simulink model "scara_2015a_dSpace"  (R2018b)
settings: Solver=ode1  StartTime=0.0  StopTime=inf  FixedStep=0.001  RelTol=1e-3
PostLoadFcn:
  | , if any(exist('dsrtsu_mdlpostloadfcn', 'file') == [2, 3, 6]), try dsrtsu_mdlpostloadfcn('Execute', bdroot); catch fprintf('Error in PostLoadFcn (dsrtsu_mdlpostloadfcn) for model "%s":\n %s\n', bdroot, lasterr); end, end,
libraries: rtilib1104 x9, simulink x5, simulink_extras x4
settings Model: DSRTSU_INTERNAL_RTI_VER=460  DSRTSU_INTERNAL_RTI_TYPE=rti1104  DSRTSU_INTERNAL_RTIFPGA=50  Creator=Bartlomiej Mroz  LastModifiedBy=Bartlomiej Mroz
settings OptimizationCC: BlockReduction=off  BooleanDataType=off  LifeSpan=inf
settings DebuggingCC: SFExecutionAtInitializationDiag=none
settings HardwareCC: ProdBitPerSizeT=32  ProdBitPerPtrDiffT=32  ProdEndianess=BigEndian  ProdWordSize=32  ProdHWDeviceType=Generic->Custom  TargetIntDivRoundTo=Zero  TargetEndianess=BigEndian  TargetHWDeviceType=Generic->Custom
settings RTWCC: SystemTargetFile=rti1104.tlc  MakeCommand=make_rti  TemplateMakefile=rti1104.tmf  Description=dSPACE DS1104 Hardware Platform
settings CodeAppCC: StateflowObjectComments=on
settings STFCustomTargetCC: ParMdlRefBuildCompliant=on  GeneratePreprocessorConditionals=Disable all  GRTInterface=on  SystemTargetFile=rti1104.tlc
settings GRTTargetCC: TargetLangStandard=C89/C90 (ANSI)  CompOptLevelCompliant=off  ConcurrentExecutionCompliant=off  GeneratePreprocessorConditionals=Disable all  CombineOutputUpdateFcns=off  MatFileLogging=off  CPPClassGenCompliant=off  GRTInterface=on  UseToolchainInfoCompliant=off  ExtModeMexFile=noextcomm

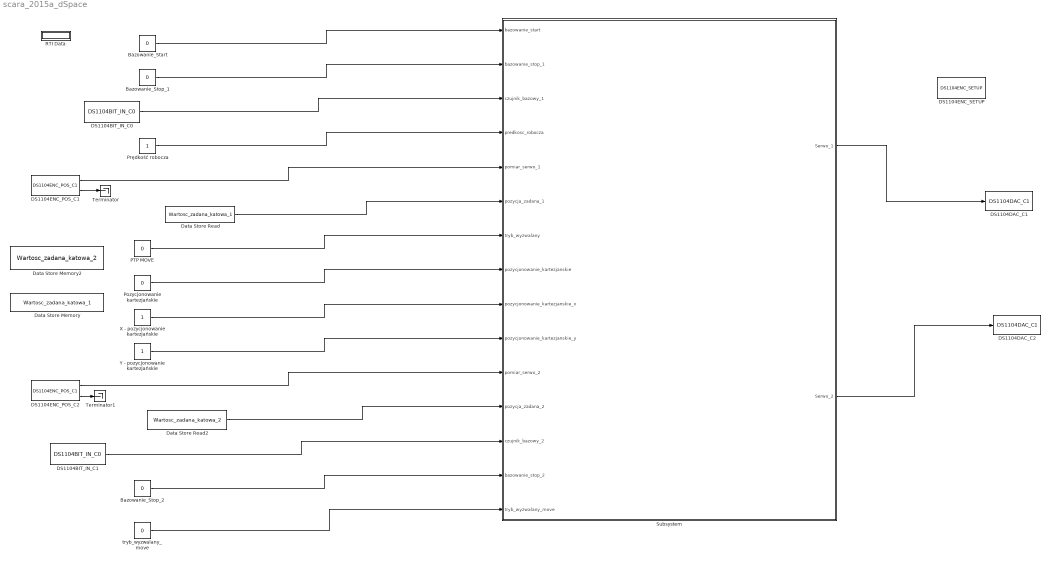
== system scara_2015a_dSpace ==
  " Bazowanie_Stop_1" : Constant  Value=0
  " Bazowanie_Stop_2" : Constant  Value=0
  " tryb_wyzwalany_move" : Constant  Value=0
  Bazowanie_Start : Constant  Value=0
  DS1104BIT_IN_C0 : rtilib1104/DS1104 MASTER PPC/DS1104BIT_IN_C0  ChannelNo=0  Reserved1=[]  Reserved2=[]  Reserved3=[]  Reserved4=[]  DialogFcn=gui1104bit_in  UnitName={'DS1104BIT_IN_C'}  UnitValues={ 0 }  DSProperties=struct('RTI',struct('Version',uint32(1),'BlockType',struct('isSLSource',uint8(1),'isSLSink',uint8(0),'isHWSource',uint8(1),'isHWSink',uint8(0),'isSetup',uint8(0),'isInline',uint8(1),'isNonInline',uint8(0),'isInterrupt',uint8(0),'isChannelwise',uint8(1)),'IOBoardType','DS1104MASTER','UnitType','BIT','Identifier','BITINCH','DialogType','ML','BlockSet','NONE','SlaveProcessor','NONE'))
  DS1104BIT_IN_C1 : rtilib1104/DS1104 MASTER PPC/DS1104BIT_IN_C0  ChannelNo=1  Reserved1=[]  Reserved2=[]  Reserved3=[]  Reserved4=[]  DialogFcn=gui1104bit_in  UnitName={'DS1104BIT_IN_C'}  UnitValues={1}  DSProperties=struct('RTI',struct('Version',uint32(1),'BlockType',struct('isSLSource',uint8(1),'isSLSink',uint8(0),'isHWSource',uint8(1),'isHWSink',uint8(0),'isSetup',uint8(0),'isInline',uint8(1),'isNonInline',uint8(0),'isInterrupt',uint8(0),'isChannelwise',uint8(1)),'IOBoardType','DS1104MASTER','UnitType','BIT','Identifier','BITINCH','DialogType','ML','BlockSet','NONE','SlaveProcessor','NONE'))
  DS1104DAC_C1 : rtilib1104/DS1104 MASTER PPC/DS1104DAC_C1  ChannelNo=1  InitValue=0  TermMode=1  TermValue=0  Reserved1=[]  Reserved2=[]  Reserved3=[]  Reserved4=[]  DialogFcn=gui1104dac  UnitName={ 'DS1104DAC_C'}  UnitValues={ 1 }  DSProperties=struct('RTI',struct('Version',uint32(1),'BlockType',struct('isSLSource',uint8(0),'isSLSink',uint8(1),'isHWSource',uint8(0),'isHWSink',uint8(1),'isSetup',uint8(0),'isInline',uint8(1),'isNonInline',uint8(0),'isInterrupt',uint8(0),'isChannelwise',uint8(1)),'IOBoardType','DS1104MASTER','UnitType','DAC','Identifier','DAC','DialogType','ML','BlockSet','NONE','SlaveProcessor','NONE'))
  DS1104DAC_C2 : rtilib1104/DS1104 MASTER PPC/DS1104DAC_C1  ChannelNo=2  InitValue=0  TermMode=1  TermValue=0  Reserved1=[]  Reserved2=[]  Reserved3=[]  Reserved4=[]  DialogFcn=gui1104dac  UnitName={ 'DS1104DAC_C'}  UnitValues={2}  DSProperties=struct('RTI',struct('Version',uint32(1),'BlockType',struct('isSLSource',uint8(0),'isSLSink',uint8(1),'isHWSource',uint8(0),'isHWSink',uint8(1),'isSetup',uint8(0),'isInline',uint8(1),'isNonInline',uint8(0),'isInterrupt',uint8(0),'isChannelwise',uint8(1)),'IOBoardType','DS1104MASTER','UnitType','DAC','Identifier','DAC','DialogType','ML','BlockSet','NONE','SlaveProcessor','NONE'))
  DS1104ENC_POS_C1 : rtilib1104/DS1104 MASTER PPC/DS1104ENC_POS_C1  ChannelNo=1  PosValue=0  Reserved1=[]  Reserved2=[]  Reserved3=[]  Reserved4=[]  DialogFcn=gui1104enc_pos  UnitName={'DS1104ENC_POS_C'}  UnitValues={ 1 }  DSProperties=struct('RTI',struct('Version',uint32(1),'BlockType',struct('isSLSource',uint8(1),'isSLSink',uint8(0),'isHWSource',uint8(1),'isHWSink',uint8(0),'isSetup',uint8(0),'isInline',uint8(1),'isNonInline',uint8(0),'isInterrupt',uint8(0),'isChannelwise',uint8(1)),'IOBoardType','DS1104MASTER','UnitType','ENC','Identifier','ENCPOSCH','DialogType','ML','BlockSet','NONE','SlaveProcessor','NONE'))
  DS1104ENC_POS_C2 : rtilib1104/DS1104 MASTER PPC/DS1104ENC_POS_C1  ChannelNo=2  PosValue=0  Reserved1=[]  Reserved2=[]  Reserved3=[]  Reserved4=[]  DialogFcn=gui1104enc_pos  UnitName={'DS1104ENC_POS_C'}  UnitValues={2}  DSProperties=struct('RTI',struct('Version',uint32(1),'BlockType',struct('isSLSource',uint8(1),'isSLSink',uint8(0),'isHWSource',uint8(1),'isHWSink',uint8(0),'isSetup',uint8(0),'isInline',uint8(1),'isNonInline',uint8(0),'isInterrupt',uint8(0),'isChannelwise',uint8(1)),'IOBoardType','DS1104MASTER','UnitType','ENC','Identifier','ENCPOSCH','DialogType','ML','BlockSet','NONE','SlaveProcessor','NONE'))
  DS1104ENC_SETUP : rtilib1104/DS1104 MASTER PPC/DS1104ENC_SETUP  Reserved1=[]  Reserved2=[]  Reserved3=[]  Reserved4=[]  DialogFcn=gui1104enc_setup  UnitName={'DS1104ENC_SETUP'}  UnitValues={ [] }  DSProperties=struct('RTI',struct('Version',uint32(1),'BlockType',struct('isSLSource',uint8(0),'isSLSink',uint8(0),'isHWSource',uint8(0),'isHWSink',uint8(0),'isSetup',uint8(0),'isInline',uint8(1),'isNonInline',uint8(0),'isInterrupt',uint8(0),'isChannelwise',uint8(0)),'IOBoardType','DS1104MASTER','UnitType','ENC','Identifier','ENCSETUP','DialogType','ML','BlockSet','NONE','SlaveProcessor','NONE'))
      settings: SignalType=[0 0]
  Data Store Memory : DataStoreMemory  DataStoreName=Wartosc_zadana_katowa_1  ReadBeforeWriteMsg=warning  WriteAfterWriteMsg=warning  WriteAfterReadMsg=warning  ShowAdditionalParam=off
  Data Store Memory2 : DataStoreMemory  DataStoreName=Wartosc_zadana_katowa_2  ReadBeforeWriteMsg=warning  WriteAfterWriteMsg=warning  WriteAfterReadMsg=warning  ShowAdditionalParam=off
  Data Store Read : DataStoreRead  DataStoreName=Wartosc_zadana_katowa_1
  Data Store Read2 : DataStoreRead  DataStoreName=Wartosc_zadana_katowa_2
  PTP MOVE : Constant  Value=0
  "Pozycjonowanie kartezjańskie " : Constant  Value=0
  Prędkość robocza : Constant
  RTI Data : Subsystem  Tag=struct('RTIDataServer',struct('RTIDataServerVs','2','RTIModelDescription','struct(''main'',''scara_2015a'',''sub'','''',''isMp'',0)'))  LoadFcn="if exist('rtidc'), try,  rtidc('DataHostBlockClbLoad', gcbh); catch, disp(['Warning: ''LoadFcn'' for RTI Data block failed: ' lasterr]); end, end,"  mask(RTI_DATA_HOST){}
      mask help:
      | RTI Data Block.
      | This block is used by RTI to store internal model-dependent data.
      | Please keep this block on the root level of the model. Deleting this block will result in data loss.
      |
      | NEVER DELETE OR COPY THIS BLOCK!
      settings: CopyFcn="if exist('rtidc'), try,  rtidc('DataHostBlockClbCopy', gcbh); catch, disp(['Warning: ''CopyFcn'' for RTI Data block failed: ' lasterr]); end, end,"  DeleteFcn="if exist('rtidc'), try,  rtidc('DataHostBlockClbDelete', gcbh); catch, disp(['Warning: ''DeleteFcn'' for RTI Data block failed: ' lasterr]); end, end,"  ModelCloseFcn="if exist('rtidc'), try,  rtidc('DataHostBlockClbModelClose', gcbh); catch, disp(['Warning: ''ModelCloseFcn'' for RTI Data block failed: ' lasterr]); end, end,"  PreSaveFcn="if exist('rtidc'), try,  rtidc('DataHostBlockClbPreSave', gcbh); catch, disp(['Warning: ''PreSaveFcn'' for RTI Data block failed: ' lasterr]); end, end,"  PostSaveFcn="if exist('rtidc'), try,  rtidc('DataHostBlockClbPostSave', gcbh); catch, disp(['Warning: ''PostSaveFcn'' for RTI Data block failed: ' lasterr]); end, end,"  NameChangeFcn="if exist('rtidc'), try,  rtidc('DataHostBlockClbNameChange', gcbh); catch, disp(['Warning: ''NameChangeFcn'' for RTI Data block failed: ' lasterr]); end, end,"
      mask Help:
      | RTI Data Block.
      | This block is used by RTI to store internal model-dependent data.
      | Please keep this block on the root level of the model. Deleting this block will result in data loss.
      | 
      | NEVER DELETE OR COPY THIS BLOCK!
      mask Display:
      | text(0.5, 0.5, 'RTI Data', 'HorizontalAlignment', 'center');
      | plot([1 0]);
  Subsystem : Subsystem
  Terminator : Terminator
  Terminator1 : Terminator
  X - pozycjonowanie kartezjańskie : Constant
  Y - pozycjonowanie kartezjańskie : Constant
  wires:
  Bazowanie_Start/1 -> Subsystem/1(bazowanie_start)
  " Bazowanie_Stop_1"/1 -> Subsystem/2(bazowanie_stop_1)
  DS1104BIT_IN_C0/1 -> Subsystem/3(czujnik_bazowy_1)
  Prędkość robocza/1 -> Subsystem/4(predkosc_robocza)
  DS1104ENC_POS_C1/1 -> Subsystem/5(pomiar_serwo_1)
  Data Store Read/1 -> Subsystem/6(pozycja_zadana_1)
  PTP MOVE/1 -> Subsystem/7(tryb_wyzwalany)
  "Pozycjonowanie kartezjańskie "/1 -> Subsystem/8(pozycjonowanie_kartezjanskie)
  X - pozycjonowanie kartezjańskie/1 -> Subsystem/9(pozycjonowanie_kartezjanskie_x)
  Y - pozycjonowanie kartezjańskie/1 -> Subsystem/10(pozycjonowanie_kartezjanskie_y)
  DS1104ENC_POS_C2/1 -> Subsystem/11(pomiar_serwo_2)
  Data Store Read2/1 -> Subsystem/12(pozycja_zadana_2)
  DS1104BIT_IN_C1/1 -> Subsystem/13(czujnik_bazowy_2)
  Subsystem/1(Serwo_1) -> DS1104DAC_C1/1
  Subsystem/2(Serwo_2) -> DS1104DAC_C2/1
  DS1104ENC_POS_C1/2 -> Terminator/1
  DS1104ENC_POS_C2/2 -> Terminator1/1
  " Bazowanie_Stop_2"/1 -> Subsystem/14(bazowanie_stop_2)
  " tryb_wyzwalany_move"/1 -> Subsystem/15(tryb_wyzwalany_move)

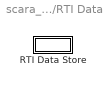
== system scara_2015a_dSpace/RTI Data ==
  RTI Data Store : Subsystem  Tag="struct('private',struct('version',struct('dsVer',uint32(2),'dsVerCreation',uint32(2),'RTI',struct('ver','7.4','type','RTI1104')),'access',struct('type','Model','isPerm',1,'created',['05-Jun-2020 16:45:06'],'modified',['05-Jun-2020 18:24:45'],'location','')),'public',struct('main',struct('data',[]),'sub',struct('name',{{'scara_2015a'}},'data',{{struct('TH',struct('thTaskInfo',struct('taskType',{'TIMER','HWINT','TMRINT','SWINT','GLINT'},'tasksNumOf',{1,0,0,0,0},'srcIds',{{'TIMERA'},{},{},{},{}},'taskNames',{{['Timer Task 1']},{},{},{},{}})),'th_tc',struct('dataType','TASK','taskGroupId','','taskGroupList',{{}},'taskSchedulingPolicy','FCFS','taskType','TIMER','blkh',-1,'srcId','TIMERA','srcSgnName',['Timer A interrupt'],'srcCpuName','','taskName',['Timer Task 1  [0.001] s'],'taskNameDisplayExt','','smplTime',0.001,'smplTimeOffs',0,'hasFixedPriority',0,'priority',1,'hasFixedOvc',0,'ovcType',1,'ovcMax',1),'tc_th',struct('dataType','TASK','taskGroupId','','taskGroupList',{{}},'taskSchedulingPolicy','FCFS','taskType','TIMER','blkh',-1,'srcId','TIMERA','srcSgnName',['Timer A interrupt'],'srcCpuName','','taskName',['Timer Task 1  [0.001] s'],'taskNameDisplayExt','','smplTime',0.001,'smplTimeOffs',0,'hasFixedPriority',0,'priority',1,'hasFixedOvc',0,'ovcType',1,'ovcMax',1))}})))"  mask(RTI_DATA_STORE){}
      mask help:
      | RTI Data Store Block. This block is used by RTI to store internal model dependent data. Deleting this block will result in data loss.
      |
      | NEVER DELETE, COPY, OR MODIFY THIS BLOCK!
      mask Help:
      | RTI Data Store Block. This block is used by RTI to store internal model dependent data. Deleting this block will result in data loss.
      | 
      | NEVER DELETE, COPY, OR MODIFY THIS BLOCK!
      mask Display: text(0.5, 0.5, ' ', 'HorizontalAlignment', 'center');

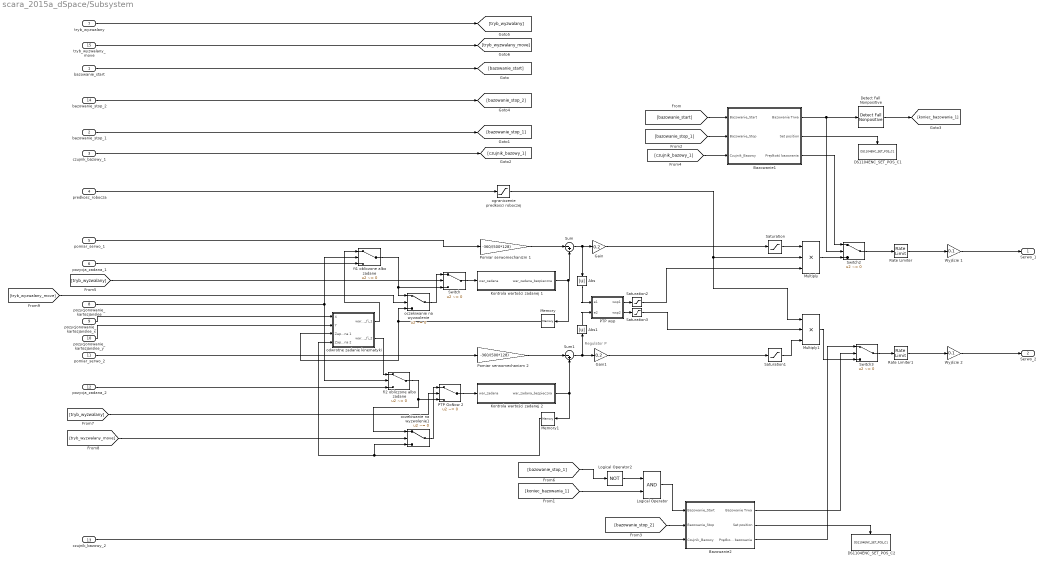
== system scara_2015a_dSpace/Subsystem ==
  note: Regulator P
  bazowanie_start : Inport
  bazowanie_stop_1 : Inport  Port=2
  czujnik_bazowy_1 : Inport  Port=3
  predkosc_robocza : Inport  Port=4
  pomiar_serwo_1 : Inport  Port=5
  pozycja_zadana_1 : Inport  Port=6
  tryb_wyzwalany : Inport  Port=7
  pozycjonowanie_kartezjanskie : Inport  Port=8
  pozycjonowanie_kartezjanskie_x : Inport  Port=9
  pozycjonowanie_kartezjanskie_y : Inport  Port=10
  pomiar_serwo_2 : Inport  Port=11
  pozycja_zadana_2 : Inport  Port=12
  czujnik_bazowy_2 : Inport  Port=13
  bazowanie_stop_2 : Inport  Port=14
  tryb_wyzwalany_move : Inport  Port=15
  Abs : Abs
  Abs1 : Abs
  Bazowanie1 : Subsystem
  Bazowanie2 : Subsystem
  DS1104ENC_SET_POS_C1 : rtilib1104/DS1104 MASTER PPC/DS1104ENC_SET_POS_C1  ChannelNo=1  PosValue=0  Reserved1=[]  Reserved2=[]  Reserved3=[]  Reserved4=[]  DialogFcn=gui1104enc_set_pos  UnitName={'DS1104ENC_SET_POS_C'}  UnitValues={ 1 }  DSProperties=struct('RTI',struct('Version',uint32(1),'BlockType',struct('isSLSource',uint8(0),'isSLSink',uint8(1),'isHWSource',uint8(0),'isHWSink',uint8(1),'isSetup',uint8(0),'isInline',uint8(1),'isNonInline',uint8(0),'isInterrupt',uint8(0),'isChannelwise',uint8(1)),'IOBoardType','DS1104MASTER','UnitType','ENC','Identifier','ENCRESET','DialogType','ML','BlockSet','NONE','SlaveProcessor','NONE'))
  DS1104ENC_SET_POS_C2 : rtilib1104/DS1104 MASTER PPC/DS1104ENC_SET_POS_C1  ChannelNo=2  PosValue=0  Reserved1=[]  Reserved2=[]  Reserved3=[]  Reserved4=[]  DialogFcn=gui1104enc_set_pos  UnitName={'DS1104ENC_SET_POS_C'}  UnitValues={2}  DSProperties=struct('RTI',struct('Version',uint32(1),'BlockType',struct('isSLSource',uint8(0),'isSLSink',uint8(1),'isHWSource',uint8(0),'isHWSink',uint8(1),'isSetup',uint8(0),'isInline',uint8(1),'isNonInline',uint8(0),'isInterrupt',uint8(0),'isChannelwise',uint8(1)),'IOBoardType','DS1104MASTER','UnitType','ENC','Identifier','ENCRESET','DialogType','ML','BlockSet','NONE','SlaveProcessor','NONE'))
  Detect Fall Nonpositive : simulink/Logic and Bit Operations/Detect Fall Nonpositive  vinit=0  OutDataTypeStr=boolean
      settings: SourceProductName=Simulink  SourceProductBaseCode=SL
  Gain : Gain  Gain=0.2
  Gain1 : Gain  Gain=0.2
  "Kontrola wartości zadanej 1 " : Subsystem
  Kontrola wartości zadanej 2 : Subsystem
  Logical Operator : Logic  AllPortsSameDT=off  OutDataTypeStr=boolean
  Logical Operator2 : Logic  Operator=NOT  AllPortsSameDT=off  OutDataTypeStr=boolean
  Memory : Memory
  Memory1 : Memory
  Multiply : Product  Inputs=3
  Multiply1 : Product  Inputs=3
  PTP GoNow 2 : Switch  Criteria=u2 ~= 0
  "PTP wsp " : MATLAB Function  TreatAsAtomicUnit=on
  Pomiar serwomechanizm 1 : Gain  Gain=-360/(500*128)
  Pomiar serwomechanizm 2 : Gain  Gain=-360/(500*128)
  Rate Limiter : RateLimiter  RisingSlewLimit=50  FallingSlewLimit=-50  SampleTimeMode=inherited
  Rate Limiter1 : RateLimiter  RisingSlewLimit=50  FallingSlewLimit=-50  SampleTimeMode=inherited
  Saturation : Saturate  UpperLimit=3  LowerLimit=-3
  Saturation1 : Saturate  UpperLimit=3  LowerLimit=-3
  Saturation2 : Saturate  UpperLimit=1  LowerLimit=0
  Saturation3 : Saturate  UpperLimit=1  LowerLimit=0
  Sum : Sum  Inputs=|-+
  Sum1 : Sum  Inputs=|-+
  Switch : Switch  Criteria=u2 ~= 0
  Switch2 : Switch  Criteria=u2 ~= 0
  Switch3 : Switch  Criteria=u2 ~= 0
  Wyjście 1 : Gain  Gain=0.1
  Wyjście 2 : Gain  Gain=0.1
  fi1 obliczone albo zadane : Switch  Criteria=u2 ~= 0
  fi2 obliczone albo zadane : Switch  Criteria=u2 ~= 0
  oczekiwanie na wyzwolenie : Switch  Criteria=u2 ~= 0
  oczekiwanie na wyzwolenie1 : Switch  Criteria=u2 ~= 0
  odwrotne zadanie kinematyki : Subsystem
  ograniczenie predkosci roboczej : Saturate  UpperLimit=1  LowerLimit=0.05
  Serwo_1 : Outport
  Serwo_2 : Outport  Port=2
  wires:
  Bazowanie1/3(Prędkość bazowania) -> Switch2/1
  [bazowanie_start] -> Bazowanie1/1(Bazowanie_Start)
  Kontrola wartości zadanej 2/1(war_zadana_bezpieczna) -> Memory1/1, Sum1/2
  [bazowanie_stop_1] -> Bazowanie1/2("Bazowanie_Stop ")
  pozycjonowanie_kartezjanskie/1 -> fi1 obliczone albo zadane/2, fi2 obliczone albo zadane/2
  Bazowanie1/1("Bazowanie Trwa ") -> Detect Fall Nonpositive/1, Switch2/2
  Multiply/1 -> Switch2/3
  Gain1/1 -> Saturation1/1
  Logical Operator/1 -> Bazowanie2/1(Bazowanie_Start)
  Sum/1 -> Abs/1, Gain/1
  ograniczenie predkosci roboczej/1 -> Multiply/2, Multiply1/1
  [bazowanie_stop_2] -> Bazowanie2/2("Bazowanie_Stop ")
  czujnik_bazowy_2/1 -> Bazowanie2/3(Czujnik_Bazowy)
  pomiar_serwo_2/1 -> Pomiar serwomechanizm 2/1
  Gain/1 -> Saturation/1
  "Kontrola wartości zadanej 1 "/1(war_zadana_bezpieczna) -> Memory/1, Sum/2
  Bazowanie2/2("Set position ") -> DS1104ENC_SET_POS_C2/Trigger
  Sum1/1 -> Gain1/1, Abs1/1
  fi1 obliczone albo zadane/1 -> oczekiwanie na wyzwolenie/1, Switch/3
  Saturation/1 -> Multiply/1
  Rate Limiter1/1 -> Wyjście 2/1
  Pomiar serwomechanizm 1/1 -> Sum/1
  pomiar_serwo_1/1 -> Pomiar serwomechanizm 1/1
  predkosc_robocza/1 -> ograniczenie predkosci roboczej/1
  "PTP wsp "/2(wsp2) -> Saturation3/1
  Wyjście 1/1 -> Serwo_1/1
  pozycjonowanie_kartezjanskie_y/1 -> odwrotne zadanie kinematyki/2(Y)
  Pomiar serwomechanizm 2/1 -> Sum1/1
  fi2 obliczone albo zadane/1 -> PTP GoNow 2/3, oczekiwanie na wyzwolenie1/1
  Wyjście 2/1 -> Serwo_2/1
  Bazowanie2/3(Prędkość bazowania) -> Switch3/1
  PTP GoNow 2/1 -> Kontrola wartości zadanej 2/1(war_zadana)
  odwrotne zadanie kinematyki/2(war_zadana_fi_2) -> fi2 obliczone albo zadane/1
  Switch3/1 -> Rate Limiter1/1
  Bazowanie2/1("Bazowanie Trwa ") -> Switch3/2
  Memory/1 -> oczekiwanie na wyzwolenie/3, odwrotne zadanie kinematyki/3(Zapamiętana zadana 1)
  Rate Limiter/1 -> Wyjście 1/1
  Switch2/1 -> Rate Limiter/1
  odwrotne zadanie kinematyki/1(war_zadana_fi_1) -> fi1 obliczone albo zadane/1
  bazowanie_stop_1/1 -> [bazowanie_stop_1]
  Multiply1/1 -> Switch3/3
  "PTP wsp "/1(wsp1) -> Saturation2/1
  bazowanie_start/1 -> [bazowanie_start]
  pozycja_zadana_1/1 -> fi1 obliczone albo zadane/3
  Bazowanie1/2("Set position ") -> DS1104ENC_SET_POS_C1/Trigger
  pozycja_zadana_2/1 -> fi2 obliczone albo zadane/3
  pozycjonowanie_kartezjanskie_x/1 -> odwrotne zadanie kinematyki/1(X)
  Abs/1 -> "PTP wsp "/1(e1)
  Abs1/1 -> "PTP wsp "/2(e2)
  Saturation3/1 -> Multiply1/2
  Saturation1/1 -> Multiply1/3
  Saturation2/1 -> Multiply/3
  czujnik_bazowy_1/1 -> [czujnik_bazowy_1]
  [czujnik_bazowy_1] -> Bazowanie1/3(Czujnik_Bazowy)
  Detect Fall Nonpositive/1 -> [koniec_bazowania_1]
  bazowanie_stop_2/1 -> [bazowanie_stop_2]
  [bazowanie_stop_1] -> Logical Operator2/1
  Logical Operator2/1 -> Logical Operator/1
  [koniec_bazowania_1] -> Logical Operator/2
  Switch/1 -> "Kontrola wartości zadanej 1 "/1(war_zadana)
  oczekiwanie na wyzwolenie/1 -> Switch/1
  Memory1/1 -> odwrotne zadanie kinematyki/4(Zapamiętna zadana 2), oczekiwanie na wyzwolenie1/3
  oczekiwanie na wyzwolenie1/1 -> PTP GoNow 2/1
  tryb_wyzwalany/1 -> [tryb_wyzwalany]
  tryb_wyzwalany_move/1 -> [tryb_wyzwalany_move]
  [tryb_wyzwalany] -> Switch/2
  [tryb_wyzwalany] -> PTP GoNow 2/2
  [tryb_wyzwalany_move] -> oczekiwanie na wyzwolenie1/2
  [tryb_wyzwalany_move] -> oczekiwanie na wyzwolenie/2

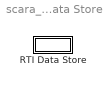
== system scara_2015a_dSpace/RTI Data/RTI Data Store ==
  RTI Data Store : Subsystem  mask(RTI_DATA_STORE){}
      mask help:
      | RTI Data Store Block. This block is used by RTI to store internal model dependent data. Deleting this block will result in data loss.
      |
      | NEVER DELETE, COPY, OR MODIFY THIS BLOCK!
      mask Help:
      | RTI Data Store Block. This block is used by RTI to store internal model dependent data. Deleting this block will result in data loss.
      | 
      | NEVER DELETE, COPY, OR MODIFY THIS BLOCK!
      mask Display: text(0.5, 0.5, ' ', 'HorizontalAlignment', 'center');

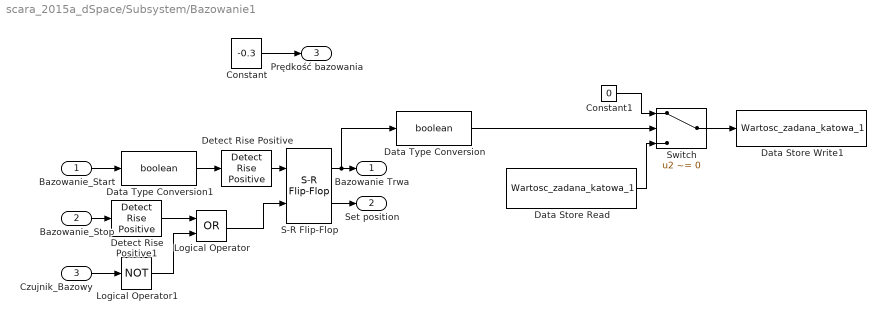
== system scara_2015a_dSpace/Subsystem/Bazowanie1 ==
  Bazowanie_Start : Inport
  "Bazowanie_Stop " : Inport  Port=2
  Czujnik_Bazowy : Inport  Port=3
  Constant : Constant  Value=-0.3
  Constant1 : Constant  Value=0
  Data Store Read : DataStoreRead  DataStoreName=Wartosc_zadana_katowa_1
  Data Store Write1 : DataStoreWrite  DataStoreName=Wartosc_zadana_katowa_1
  Data Type Conversion : DataTypeConversion  OutDataTypeStr=boolean
  Data Type Conversion1 : DataTypeConversion  OutDataTypeStr=boolean
  Detect Rise Positive : simulink/Logic and Bit Operations/Detect Rise Positive  vinit=0  OutDataTypeStr=boolean
  Detect Rise Positive1 : simulink/Logic and Bit Operations/Detect Rise Positive  vinit=0  OutDataTypeStr=boolean
  Logical Operator : Logic  Operator=OR  AllPortsSameDT=off  OutDataTypeStr=boolean
  Logical Operator1 : Logic  Operator=NOT  AllPortsSameDT=off  OutDataTypeStr=boolean
  S-R Flip-Flop : simulink_extras/Flip Flops/S-R Flip-Flop  initial_condition=0
  Switch : Switch  Criteria=u2 ~= 0
  "Bazowanie Trwa " : Outport
  "Set position " : Outport  Port=2
  Prędkość bazowania : Outport  Port=3
  wires:
  "Bazowanie_Stop "/1 -> Detect Rise Positive1/1
  Czujnik_Bazowy/1 -> Logical Operator1/1
  Logical Operator1/1 -> Logical Operator/2
  Logical Operator/1 -> S-R Flip-Flop/2
  Bazowanie_Start/1 -> Data Type Conversion1/1
  S-R Flip-Flop/1 -> Data Type Conversion/1, "Bazowanie Trwa "/1
  S-R Flip-Flop/2 -> "Set position "/1
  Constant/1 -> Prędkość bazowania/1
  Switch/1 -> Data Store Write1/1
  Constant1/1 -> Switch/1
  Data Store Read/1 -> Switch/3
  Data Type Conversion/1 -> Switch/2
  Detect Rise Positive1/1 -> Logical Operator/1
  Data Type Conversion1/1 -> Detect Rise Positive/1
  Detect Rise Positive/1 -> S-R Flip-Flop/1

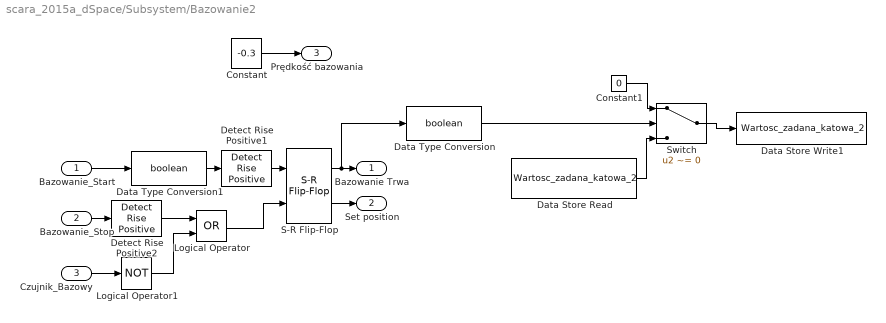
== system scara_2015a_dSpace/Subsystem/Bazowanie2 ==
  Bazowanie_Start : Inport
  "Bazowanie_Stop " : Inport  Port=2
  Czujnik_Bazowy : Inport  Port=3
  Constant : Constant  Value=-0.3
  Constant1 : Constant  Value=0
  Data Store Read : DataStoreRead  DataStoreName=Wartosc_zadana_katowa_2
  Data Store Write1 : DataStoreWrite  DataStoreName=Wartosc_zadana_katowa_2
  Data Type Conversion : DataTypeConversion  OutDataTypeStr=boolean
  Data Type Conversion1 : DataTypeConversion  OutDataTypeStr=boolean
  Detect Rise Positive1 : simulink/Logic and Bit Operations/Detect Rise Positive  vinit=0  OutDataTypeStr=boolean
  Detect Rise Positive2 : simulink/Logic and Bit Operations/Detect Rise Positive  vinit=0  OutDataTypeStr=boolean
  Logical Operator : Logic  Operator=OR  AllPortsSameDT=off  OutDataTypeStr=boolean
  Logical Operator1 : Logic  Operator=NOT  AllPortsSameDT=off  OutDataTypeStr=boolean
  S-R Flip-Flop : simulink_extras/Flip Flops/S-R Flip-Flop  initial_condition=0
  Switch : Switch  Criteria=u2 ~= 0
  "Bazowanie Trwa " : Outport
  "Set position " : Outport  Port=2
  Prędkość bazowania : Outport  Port=3
  wires:
  "Bazowanie_Stop "/1 -> Detect Rise Positive2/1
  Czujnik_Bazowy/1 -> Logical Operator1/1
  Logical Operator1/1 -> Logical Operator/2
  Logical Operator/1 -> S-R Flip-Flop/2
  Bazowanie_Start/1 -> Data Type Conversion1/1
  S-R Flip-Flop/2 -> "Set position "/1
  Constant/1 -> Prędkość bazowania/1
  Data Store Read/1 -> Switch/3
  Switch/1 -> Data Store Write1/1
  Constant1/1 -> Switch/1
  S-R Flip-Flop/1 -> Data Type Conversion/1, "Bazowanie Trwa "/1
  Data Type Conversion/1 -> Switch/2
  Data Type Conversion1/1 -> Detect Rise Positive1/1
  Detect Rise Positive1/1 -> S-R Flip-Flop/1
  Detect Rise Positive2/1 -> Logical Operator/1

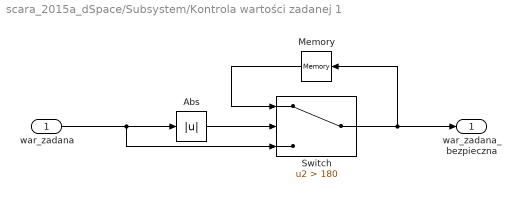
== system scara_2015a_dSpace/Subsystem/Kontrola wartości zadanej 1  ==
  war_zadana : Inport
  Abs : Abs
  Memory : Memory
  Switch : Switch  Criteria=u2 > Threshold  Threshold=180
  war_zadana_bezpieczna : Outport
  wires:
  war_zadana/1 -> Switch/3, Abs/1
  Abs/1 -> Switch/2
  Switch/1 -> Memory/1, war_zadana_bezpieczna/1
  Memory/1 -> Switch/1

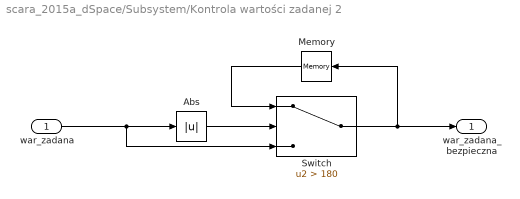
== system scara_2015a_dSpace/Subsystem/Kontrola wartości zadanej 2 ==
  war_zadana : Inport
  Abs : Abs
  Memory : Memory
  Switch : Switch  Criteria=u2 > Threshold  Threshold=180
  war_zadana_bezpieczna : Outport
  wires:
  Memory/1 -> Switch/1
  Switch/1 -> war_zadana_bezpieczna/1, Memory/1
  Abs/1 -> Switch/2
  war_zadana/1 -> Abs/1, Switch/3

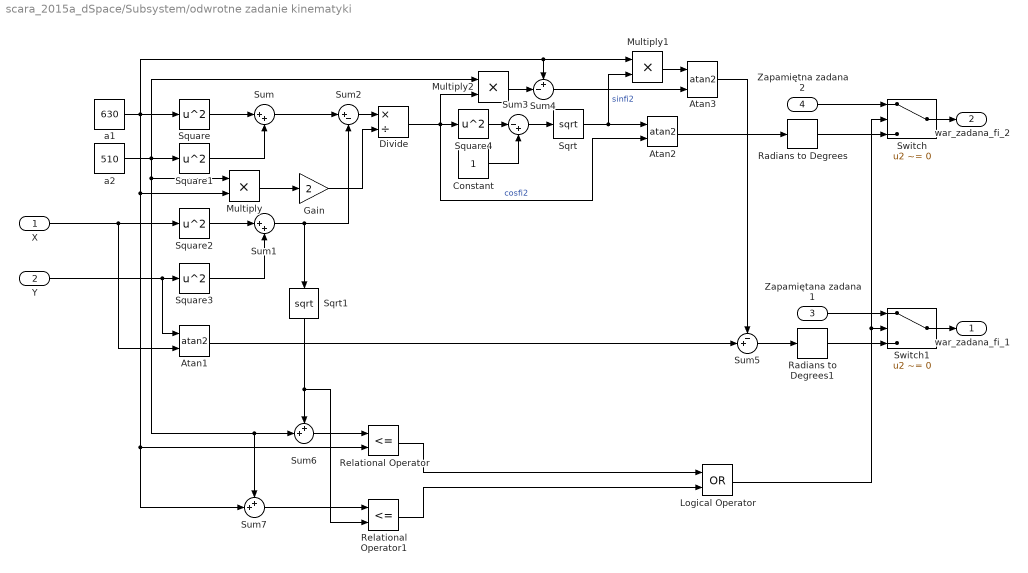
== system scara_2015a_dSpace/Subsystem/odwrotne zadanie kinematyki ==
  X : Inport
  Y : Inport  Port=2
  Zapamiętana zadana 1 : Inport  Port=3
  Zapamiętna zadana 2 : Inport  Port=4
  Atan1 : Trigonometry  Operator=atan2
  Atan2 : Trigonometry  Operator=atan2
  Atan3 : Trigonometry  Operator=atan2
  Constant : Constant
  Divide : Product  Inputs=*/
  Gain : Gain  Gain=2
  Logical Operator : Logic  Operator=OR  AllPortsSameDT=off  OutDataTypeStr=boolean
  Multiply : Product
  Multiply1 : Product
  Multiply2 : Product
  Radians to Degrees : simulink_extras/Transformations/Radians to Degrees
  Radians to Degrees1 : simulink_extras/Transformations/Radians to Degrees
  Relational Operator : RelationalOperator  Operator=<=  OutDataTypeStr=boolean  RndMeth=Simplest
  Relational Operator1 : RelationalOperator  Operator=<=  OutDataTypeStr=boolean  RndMeth=Simplest
  Sqrt : Sqrt  SaturateOnIntegerOverflow=on
  Sqrt1 : Sqrt  SaturateOnIntegerOverflow=on
  Square{,1..4} (5 alike) : Math  Operator=square  SaturateOnIntegerOverflow=on
  Sum : Sum  Inputs=|++
  Sum1 : Sum  Inputs=|++
  Sum2 : Sum  Inputs=|+-
  Sum3 : Sum  Inputs=|-+
  Sum4 : Sum  Inputs=+-|
  Sum5 : Sum  Inputs=-+|
  Sum6 : Sum  Inputs=++|
  Sum7 : Sum  Inputs=++|
  Switch : Switch  Criteria=u2 ~= 0
  Switch1 : Switch  Criteria=u2 ~= 0
  a1 : Constant  Value=630
  a2 : Constant  Value=510
  war_zadana_fi_1 : Outport
  war_zadana_fi_2 : Outport  Port=2
  wires:
  a2/1 -> Multiply2/1, Square1/1, Multiply/1, Sum7/1, Sum6/2
  X/1 -> Square2/1, Atan1/2
  Y/1 -> Atan1/1, Square3/1
  Multiply/1 -> Gain/1
  Square/1 -> Sum/1
  Square1/1 -> Sum/2
  Square2/1 -> Sum1/1
  Square3/1 -> Sum1/2
  Sum/1 -> Sum2/1
  Sum1/1 -> Sqrt1/1, Sum2/2
  Sum2/1 -> Divide/1
  Gain/1 -> Divide/2
  Divide/1 -> Multiply2/2, Atan2/2, Square4/1  "cosfi2"
  Square4/1 -> Sum3/1
  Sum3/1 -> Sqrt/1
  Constant/1 -> Sum3/2
  Sqrt/1 -> Multiply1/2, Atan2/1  "sinfi2"
  a1/1 -> Sum4/1, Multiply1/1, Square/1, Multiply/2, Sum7/2, Relational Operator/2
  Multiply2/1 -> Sum4/2
  Multiply1/1 -> Atan3/1
  Sum4/1 -> Atan3/2
  Atan1/1 -> Sum5/2
  Atan3/1 -> Sum5/1
  Atan2/1 -> Radians to Degrees/1
  Sum5/1 -> Radians to Degrees1/1
  Sum6/1 -> Relational Operator/1
  Sqrt1/1 -> Relational Operator1/2, Sum6/1
  Relational Operator/1 -> Logical Operator/1
  Relational Operator1/1 -> Logical Operator/2
  Sum7/1 -> Relational Operator1/1
  Radians to Degrees1/1 -> Switch1/3
  Radians to Degrees/1 -> Switch/3
  Switch/1 -> war_zadana_fi_2/1
  Switch1/1 -> war_zadana_fi_1/1
  Logical Operator/1 -> Switch/2, Switch1/2
  Zapamiętana zadana 1/1 -> Switch1/1
  Zapamiętna zadana 2/1 -> Switch/1

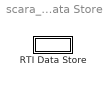
== system scara_2015a_dSpace/RTI Data/RTI Data Store/RTI Data Store ==
  RTI Data Store : Subsystem  mask(RTI_DATA_STORE){}
      mask help:
      | RTI Data Store Block. This block is used by RTI to store internal model dependent data. Deleting this block will result in data loss.
      |
      | NEVER DELETE, COPY, OR MODIFY THIS BLOCK!
      mask Help:
      | RTI Data Store Block. This block is used by RTI to store internal model dependent data. Deleting this block will result in data loss.
      | 
      | NEVER DELETE, COPY, OR MODIFY THIS BLOCK!
      mask Display: text(0.5, 0.5, ' ', 'HorizontalAlignment', 'center');

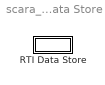
== system scara_2015a_dSpace/RTI Data/RTI Data Store/RTI Data Store/RTI Data Store ==
  RTI Data Store : Subsystem  mask(RTI_DATA_STORE){}
      mask help:
      | RTI Data Store Block. This block is used by RTI to store internal model dependent data. Deleting this block will result in data loss.
      |
      | NEVER DELETE, COPY, OR MODIFY THIS BLOCK!
      mask Help:
      | RTI Data Store Block. This block is used by RTI to store internal model dependent data. Deleting this block will result in data loss.
      | 
      | NEVER DELETE, COPY, OR MODIFY THIS BLOCK!
      mask Display: text(0.5, 0.5, ' ', 'HorizontalAlignment', 'center');

== system scara_2015a_dSpace/RTI Data/RTI Data Store/RTI Data Store/RTI Data Store/RTI Data Store ==

== matlab function scara_2015a_dSpace/Subsystem/PTP wsp  ==
  data: e1 input; wsp1 output; e2 input; wsp2 output
function [wsp1,wsp2] = fcn(e1,e2)
denum = max(e1,e2);
if ~denum
    denum = 0.01;
end
wsp1 = e1/denum;
wsp2 = e2/denum;
